simulink model "Modele_CorrecteurPD"  (R2015b)
settings: Solver=VariableStepAuto  StartTime=0.0  StopTime=10.0  RelTol=1e-3
settings Model: Creator=pt_ptsi  LastModifiedBy=pt_ptsi

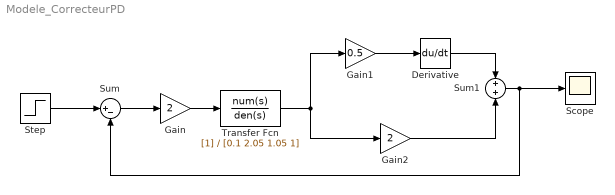
== system Modele_CorrecteurPD ==
  Derivative : Derivative
  Gain : Gain  Gain=2
  Gain1 : Gain  Gain=0.5
  Gain2 : Gain  Gain=2
  Scope : Scope
  Step : Step  Time=0  SampleTime=0
  Sum : Sum  Inputs=|+-
  Sum1 : Sum  Inputs=+|+
  Transfer Fcn : TransferFcn  Denominator=[0.1 2.05 1.05 1]
  wires:
  Gain/1 -> Transfer Fcn/1
  Sum/1 -> Gain/1
  Step/1 -> Sum/1
  Gain1/1 -> Derivative/1
  Transfer Fcn/1 -> Gain1/1, Gain2/1
  Derivative/1 -> Sum1/1
  Gain2/1 -> Sum1/2
  Sum1/1 -> Scope/1, Sum/2
